simulink model "convController"  (R2015a)
settings: Solver=ode45  StartTime=0.0  StopTime=10.0  RelTol=1e-3
values from neighbouring files (symbols this model uses):
  B = [B zeros(n_states,1)]    [OnlyRigidBody.m]
  C = [C;Cdiff]    [OnlyRigidBody.m]
  D = [D;Ddiff]    [OnlyRigidBody.m]
undefined symbols (not defined in the file or in its folder): A
settings Model: Creator=anatole  LastModifiedBy=anatole

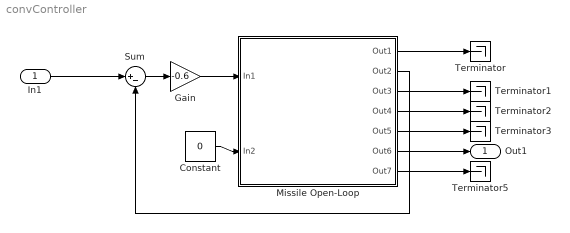
== system convController ==
  In1 : Inport
  Constant : Constant  Value=0
  Gain : Gain  Gain=-0.6
  Missile Open-Loop : Subsystem
      mask Display:
      | port_label('input', 1, '\theta_T','texmode','on')
      | port_label('input', 2, 'a_{zref}','texmode','on')
      | 
      | port_label('output', 1, '\alpha','texmode','on')
      | port_label('output', 2, 'q','texmode','on')
      | port_label('output', 3, 'a_z','texmode','on')
      | port_label('output', 4, 'a_{zIMU}','texmode','on')
      | port_label('output', 5, 'a_{zref}','texmode','on')
      | port_label('output', 6, 'a_{zref}-a_z','texmode','on')
      | port_label('output', 7, '\theta_T','texmode','on')
  Sum : Sum  Inputs=|+-
  Terminator{,1..3,5} (5 alike) : Terminator
  Out1 : Outport
  wires:
  Constant/1 -> Missile Open-Loop/2(In2)
  Gain/1 -> Missile Open-Loop/1(In1)
  Sum/1 -> Gain/1
  Missile Open-Loop/2(Out2) -> Sum/2
  In1/1 -> Sum/1
  Missile Open-Loop/1(Out1) -> Terminator/1
  Missile Open-Loop/3(Out3) -> Terminator1/1
  Missile Open-Loop/4(Out4) -> Terminator2/1
  Missile Open-Loop/5(Out5) -> Terminator3/1
  Missile Open-Loop/7(Out7) -> Terminator5/1
  Missile Open-Loop/6(Out6) -> Out1/1

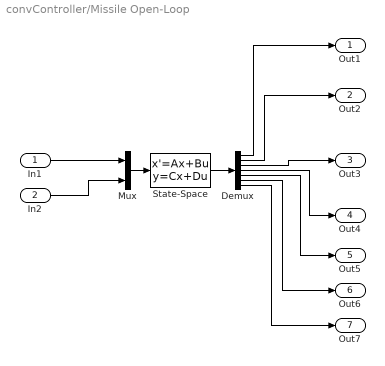
== system convController/Missile Open-Loop ==
  In1 : Inport
  In2 : Inport  Port=2
  Demux : Demux  Outputs=7
  Mux : Mux  Inputs=2
  State-Space : StateSpace  A=A  B=B  C=C  D=D  X0=0
  Out1 : Outport
  Out2 : Outport  Port=2
  Out3 : Outport  Port=3
  Out4 : Outport  Port=4
  Out5 : Outport  Port=5
  Out6 : Outport  Port=6
  Out7 : Outport  Port=7
  wires:
  In1/1 -> Mux/1
  In2/1 -> Mux/2
  Mux/1 -> State-Space/1
  State-Space/1 -> Demux/1
  Demux/3 -> Out3/1
  Demux/2 -> Out2/1
  Demux/4 -> Out4/1
  Demux/5 -> Out5/1
  Demux/1 -> Out1/1
  Demux/6 -> Out6/1
  Demux/7 -> Out7/1
